simulink model "cruise_control"  (R2020b)
settings: Solver=VariableStepAuto  StartTime=0.0  StopTime=120  RelTol=1e-3
undefined symbols (not defined in the file): b, m
settings Model: Creator=lenovo  LastModifiedBy=lenovo

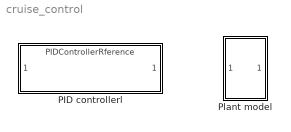
== system cruise_control ==
  PID controllerl : ModelReference  ModelNameDialog=PIDControllerRference.slx  SimulationMode=Normal  ModelReferenceVersion=1.1
  Plant model : Subsystem

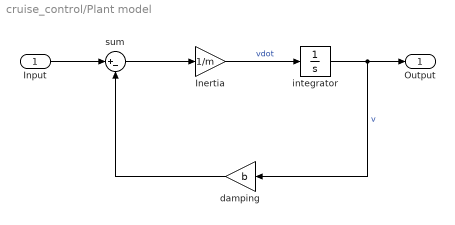
== system cruise_control/Plant model ==
  Input : Inport
  Inertia : Gain  Gain=1/m
  damping : Gain  Gain=b
  integrator : Integrator
  sum : Sum  Inputs=|+-
  Output : Outport
  wires:
  integrator/1 -> Output/1, damping/1  "v"
  sum/1 -> Inertia/1
  Inertia/1 -> integrator/1  "vdot"
  Input/1 -> sum/1
  damping/1 -> sum/2
